simulink model "P9s"  (R2015b)
settings: Solver=VariableStepAuto  StartTime=0.0  StopTime=7  RelTol=1e-3
settings Model: Creator=xmax1946  LastModifiedBy=xmax1946

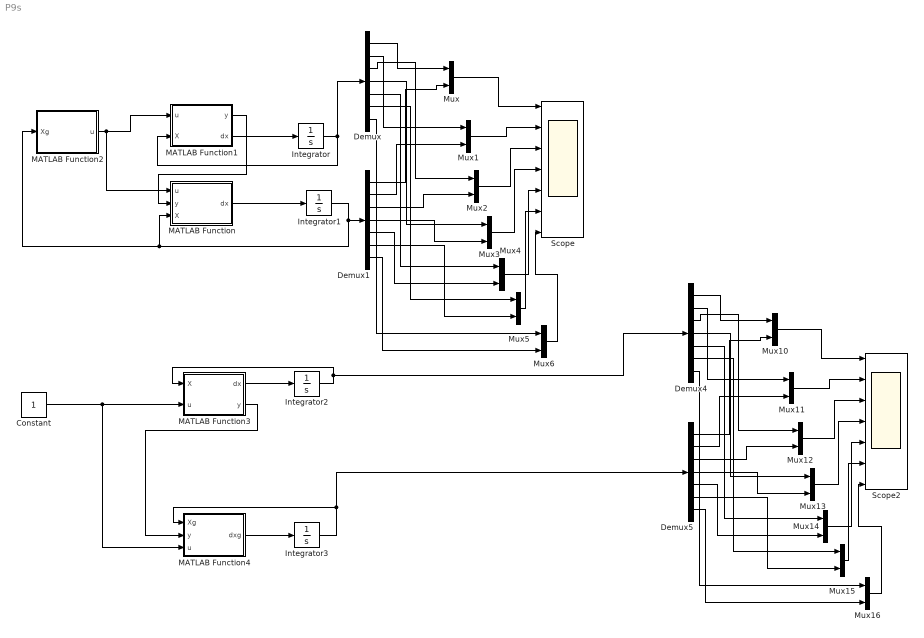
== system P9s ==
  Constant : Constant
  Demux{,1,4..5} (4 alike) : Demux  Outputs=7
  Integrator : Integrator  InitialCondition=[.1;.1;.1;.1;.1;.1;.1]  IgnoreLimit=on
  Integrator1 : Integrator  InitialCondition=[.2;.2;.2;.2;.2;.2;.2]
  Integrator2 : Integrator  InitialCondition=[.1;.1;.1;.1;.1;.1;.1]
  Integrator3 : Integrator  InitialCondition=[.2;.2;.2;.2;.2;.2;.2]
  MATLAB Function : MATLAB Function  TreatAsAtomicUnit=on
  MATLAB Function1 : MATLAB Function  TreatAsAtomicUnit=on
  MATLAB Function2 : MATLAB Function  TreatAsAtomicUnit=on
  MATLAB Function3 : MATLAB Function  TreatAsAtomicUnit=on
  MATLAB Function4 : MATLAB Function  TreatAsAtomicUnit=on
  Mux{,1..6,10..16} (14 alike) : Mux  Inputs=2
  Scope : Scope  NumInputPorts=7
  Scope2 : Scope  NumInputPorts=7
  wires:
  MATLAB Function2/1(u) -> MATLAB Function/1(u), MATLAB Function1/1(u)
  MATLAB Function/1(dx) -> Integrator1/1
  MATLAB Function1/2(dx) -> Integrator/1
  Integrator/1 -> MATLAB Function1/2(X), Demux/1
  Integrator1/1 -> Demux1/1, MATLAB Function2/1(Xg), MATLAB Function/3(X)
  MATLAB Function1/1(y) -> MATLAB Function/2(y)
  Demux/1 -> Mux/1
  Demux1/1 -> Mux/2
  Mux/1 -> Scope/1
  Demux/2 -> Mux1/1
  Demux1/2 -> Mux1/2
  Demux/3 -> Mux2/1
  Demux1/3 -> Mux2/2
  Mux1/1 -> Scope/2
  Mux2/1 -> Scope/3
  Demux/4 -> Mux3/1
  Demux1/4 -> Mux3/2
  Demux/5 -> Mux4/1
  Demux1/5 -> Mux4/2
  Demux/6 -> Mux5/1
  Demux1/6 -> Mux5/2
  Demux1/7 -> Mux6/2
  Mux3/1 -> Scope/4
  Mux4/1 -> Scope/5
  Mux5/1 -> Scope/6
  Mux6/1 -> Scope/7
  MATLAB Function3/1(dx) -> Integrator2/1
  MATLAB Function4/1(dxg) -> Integrator3/1
  MATLAB Function3/2(y) -> MATLAB Function4/2(y)
  Constant/1 -> MATLAB Function4/3(u), MATLAB Function3/2(u)
  Integrator2/1 -> Demux4/1, MATLAB Function3/1(X)
  Integrator3/1 -> Demux5/1, MATLAB Function4/1(Xg)
  Demux4/1 -> Mux10/1
  Demux5/1 -> Mux10/2
  Mux10/1 -> Scope2/1
  Demux4/2 -> Mux11/1
  Demux5/2 -> Mux11/2
  Demux4/3 -> Mux12/1
  Demux5/3 -> Mux12/2
  Mux11/1 -> Scope2/2
  Mux12/1 -> Scope2/3
  Demux4/4 -> Mux13/1
  Demux5/4 -> Mux13/2
  Demux4/5 -> Mux14/1
  Demux5/5 -> Mux14/2
  Demux4/6 -> Mux15/1
  Demux5/6 -> Mux15/2
  Demux5/7 -> Mux16/2
  Mux13/1 -> Scope2/4
  Mux14/1 -> Scope2/5
  Mux15/1 -> Scope2/6
  Mux16/1 -> Scope2/7
  Demux4/7 -> Mux16/1
  Demux/7 -> Mux6/1

== matlab function P9s/MATLAB Function1 ==
  data: u input; y output; X input; dx output
function [y,dx] = fcn(u,X)
A=[-5,6,-7,1,6,-3,1;
    -3,1,-4,2,-5,7,1;
    0,0,-6,12,-14,6,1;
    0,0,0,6,-14,11,-8;
    0,0,0,7,-8,4,-8;
    0,0,0,0,0,3,-8;
    0,0,0,0,0,4,-5];
B=[3;2;1;0;0;0;0];
C=[1,-1,1,0,-1,1,-1];

dx=A*X+B*u;
y=C*X;

== matlab function P9s/MATLAB Function ==
  data: u input; y input; X input; dx output
function dx  = fcn(u,y,X)
A=[-5,6,-7,1,6,-3,1;
    -3,1,-4,2,-5,7,1;
    0,0,-6,12,-14,6,1;
    0,0,0,6,-14,11,-8;
    0,0,0,7,-8,4,-8;
    0,0,0,0,0,3,-8;
    0,0,0,0,0,4,-5];
B=[3;2;1;0;0;0;0];
C=[1,-1,1,0,-1,1,-1];

L=[57.7467;0;-37.7467;-40.3067;0;0;0];
L=[58;0;-38;-40;0;0;0];
dx=A*X+B*u+(L*(y-C*X));

== matlab function P9s/MATLAB Function2 ==
  data: u output; Xg input
function u = fcn(Xg)
K=[ 7876504266813290642357807344911946971078006407513/285449538541191976211657193889899027276549324800, -5387384290734095850786359727540078631041915420927/142724769270595988105828596944949513638274662400, 453626891665044071127847316956831207346822709293/35681192317648997026457149236237378409568665600, 7876504266813290642357807344911946971078006407513/285449538541191976211657193889899027276549324800, -18651272848281482343930526799992104233161837249367/285449538541191976211657193889899027276549324800, 5387384290734095850786359727540078631041915420927/142724769270595988105828596944949513638274662400, 15022257714961129774907748264337454574387255575023/285449538541191976211657193889899027276549324800];
r=1;
u=r-K*Xg;

== matlab function P9s/MATLAB Function3 ==
  data: dx output; X input; y output; u input
function [dx,y]=fcn(X,u)
A=[-5,6,-7,1,6,-3,1;
    -3,1,-4,2,-5,7,1;
    0,0,-6,12,-14,6,1;
    0,0,0,6,-14,11,-8;
    0,0,0,7,-8,4,-8;
    0,0,0,0,0,3,-8;
    0,0,0,0,0,4,-5];
B=[3;2;1;0;0;0;0];
C=[1,-1,1,0,-1,1,-1];

dx=A*X+B*u;
y=C*X;

== matlab function P9s/MATLAB Function4 ==
  data: Xg input; y input; u input; dxg output
function dxg =fcn(Xg,y,u)
A=[-5,6,-7,1,6,-3,1;
    -3,1,-4,2,-5,7,1;
    0,0,-6,12,-14,6,1;
    0,0,0,6,-14,11,-8;
    0,0,0,7,-8,4,-8;
    0,0,0,0,0,3,-8;
    0,0,0,0,0,4,-5];
B=[3;2;1;0;0;0;0];
C=[1,-1,1,0,-1,1,-1];

L=[57.7467;0;-37.7467;-40.3067;0;0;0];
% L=[58;0;-38;-40;0;0;0];

dxg=A*Xg+B*u+L*(y-C*Xg);
